simulink model "MatMul_Top"  (R2023b)
settings: Solver=VariableStepAuto  StartTime=0.0  StopTime=10.0  RelTol=1e-3
libraries: prociolib x3, socmemlib x1
settings Model: Creator=lenovo GAME  LastModifiedBy=lenovo GAME

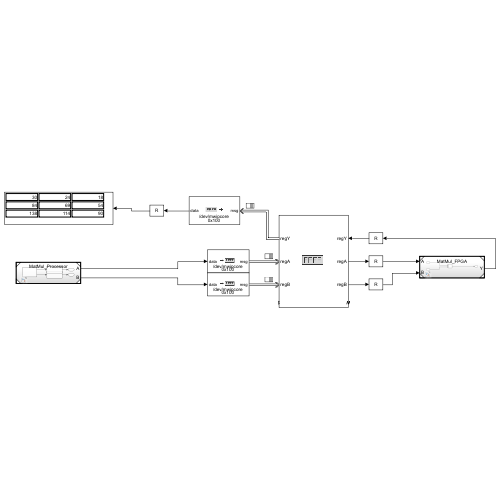
[thumbnail: Simulink's stored preview of the top-level diagram]
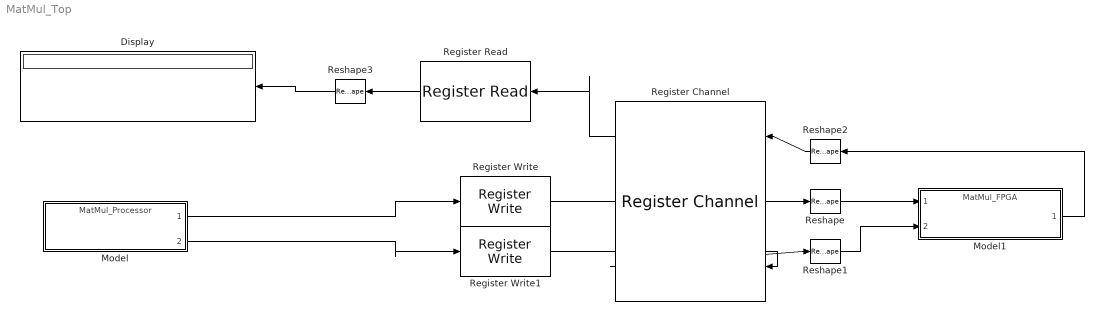
== system MatMul_Top ==
  Display : Display
  Model : ModelReference  ModelNameDialog=MatMul_Processor.slx  SimulationMode=Normal  ModelReferenceVersion=1.4
  Model1 : ModelReference  ModelNameDialog=MatMul_FPGA.slx  SimulationMode=Normal  ModelReferenceVersion=1.2
  Register Channel : socmemlib/Register Channel  RegisterTable={ 'regB', 'Write', 'fixdt(1,16,8)', '9'; 'regA', 'Write', 'fixdt(1,16,8)', '9'; 'regY', 'Read', 'fixdt(1,32,16)', '9' }  SampleTime=-1  RegTableNames={'regB' 'regA' 'regY' }  RegTableRW={'Write' 'Write' 'Read' }  RegTableDataTypes={'fixdt(1,16,8)' 'fixdt(1,16,8)' 'fixdt(1,32,16)' }  RegTableVectorSizes={'9' '9' '9' }  NumRegisters=3  RegTableDefaultValues="{'x\"0000\"' 'x\"0000\"' 'x\"0000\"' }"  RegTableDirty=0
  Register Read : prociolib/Register Read  DeviceName=/dev/mwipcore  OffsetAddress=hex2dec('0100')  OutDataTypeStr=fixdt(1,32,16)  OutputVectorSize=9  SampleTime=-1  Dummy=0
  Register Write : prociolib/Register Write  OutputSink=To output port  TunableParamName=A  RegisterName=RegA  DeviceName=/dev/mwipcore  OffsetAddress=hex2dec('100')  Dummy=0
  Register Write1 : prociolib/Register Write  OutputSink=To output port  TunableParamName=A  RegisterName=RegA  DeviceName=/dev/mwipcore  OffsetAddress=hex2dec('100')  Dummy=0
  Reshape : Reshape  OutputDimensionality=Customize  OutputDimensions=[3 3]
  Reshape1 : Reshape  OutputDimensionality=Customize  OutputDimensions=[3 3]
  Reshape2 : Reshape  OutputDimensionality=Customize  OutputDimensions=[9 1]
  Reshape3 : Reshape  OutputDimensionality=Customize  OutputDimensions=[3 3]
  wires:
  Model/1 -> Register Write/1
  Model/2 -> Register Write1/1
  Register Channel/2 -> Reshape/1
  Register Channel/1 -> Reshape1/1
  Model1/1 -> Reshape2/1
  Register Channel/3 -> Register Read/1
  Register Write1/1 -> Register Channel/1
  Register Write/1 -> Register Channel/2
  Reshape/1 -> Model1/1
  Reshape1/1 -> Model1/2
  Reshape2/1 -> Register Channel/3
  Register Read/1 -> Reshape3/1
  Reshape3/1 -> Display/1
